simulink model "single_phase_inverter_rpid"  (R2020a)
settings: Solver=VariableStepAuto  StartTime=0.0  StopTime=simlength  RelTol=1e-3
undefined symbols (not defined in the file): A, Aed, Aresd, B, Bed, Bresd, C, Ce, Cres, d, E, ki, kp, Led, simlength, Tc, Ts, w, w0
settings Model: Creator=dbagn  LastModifiedBy=dabagnara
settings DataIOCC: ReturnWorkspaceOutputs=off

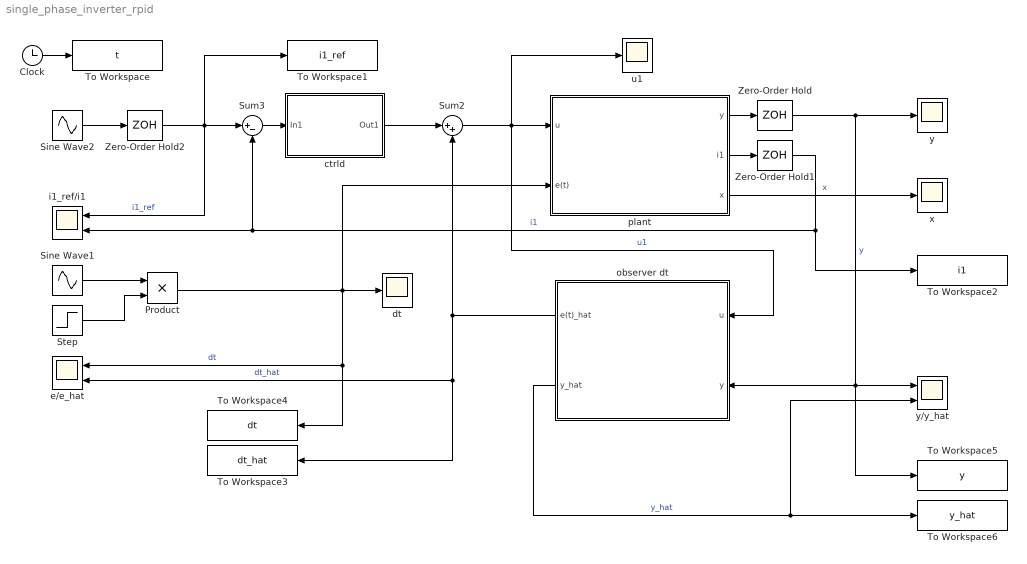
== system single_phase_inverter_rpid ==
  Clock : Clock
  Product : Product
  Sine Wave1 : Sin  Amplitude=d  Frequency=w  SampleTime=0
  Sine Wave2 : Sin  Amplitude=20  Frequency=w0  SampleTime=0
  Step : Step  Time=simlength/2  SampleTime=0
  Sum2 : Sum  Inputs=|++
  Sum3 : Sum  Inputs=|+-
  To Workspace : ToWorkspace  VariableName=t  SampleTime=Tc
      settings: MaxDataPoints=Nc
  To Workspace1 : ToWorkspace  VariableName=i1_ref  SampleTime=Tc
      settings: MaxDataPoints=Nc
  To Workspace2 : ToWorkspace  VariableName=i1  SampleTime=Tc
      settings: MaxDataPoints=Nc
  To Workspace3 : ToWorkspace  VariableName=dt_hat  SampleTime=Tc
      settings: MaxDataPoints=Nc
  To Workspace4 : ToWorkspace  VariableName=dt  SampleTime=Tc
      settings: MaxDataPoints=Nc
  To Workspace5 : ToWorkspace  VariableName=y  SampleTime=Tc
      settings: MaxDataPoints=Nc
  To Workspace6 : ToWorkspace  VariableName=y_hat  SampleTime=Tc
      settings: MaxDataPoints=Nc
  Zero-Order Hold : ZeroOrderHold  SampleTime=Ts
  Zero-Order Hold1 : ZeroOrderHold  SampleTime=Ts
  Zero-Order Hold2 : ZeroOrderHold  SampleTime=Ts
  ctrld : Subsystem
  dt : Scope
  e/e_hat : Scope  NumInputPorts=2
  i1_ref/i1 : Scope  NumInputPorts=2
  observer dt : Subsystem
  "plant " : Subsystem
  u1 : Scope
  x : Scope
  y : Scope
  y/y_hat : Scope  NumInputPorts=2
  wires:
  observer dt/2(y_hat) -> To Workspace6/1, y/y_hat/2  "y_hat"
  "plant "/1(y) -> Zero-Order Hold/1
  Product/1 -> To Workspace4/1, e/e_hat/1, dt/1, "plant "/2(e(t))  "dt"
  Sine Wave2/1 -> Zero-Order Hold2/1
  ctrld/1(Out1) -> Sum2/1
  Sum2/1 -> observer dt/1(u), "plant "/1(u), u1/1  "u1"
  "plant "/2(i1) -> Zero-Order Hold1/1
  "plant "/3(x) -> x/1  "x"
  Sum3/1 -> ctrld/1(In1)
  observer dt/1(e(t)_hat) -> Sum2/2, To Workspace3/1, e/e_hat/2  "dt_hat"
  Zero-Order Hold/1 -> To Workspace5/1, observer dt/2(y), y/y_hat/1, y/1  "y"
  Zero-Order Hold1/1 -> To Workspace2/1, Sum3/2, i1_ref/i1/2  "i1"
  Zero-Order Hold2/1 -> To Workspace1/1, Sum3/1, i1_ref/i1/1  "i1_ref"
  Sine Wave1/1 -> Product/1
  Step/1 -> Product/2
  Clock/1 -> To Workspace/1

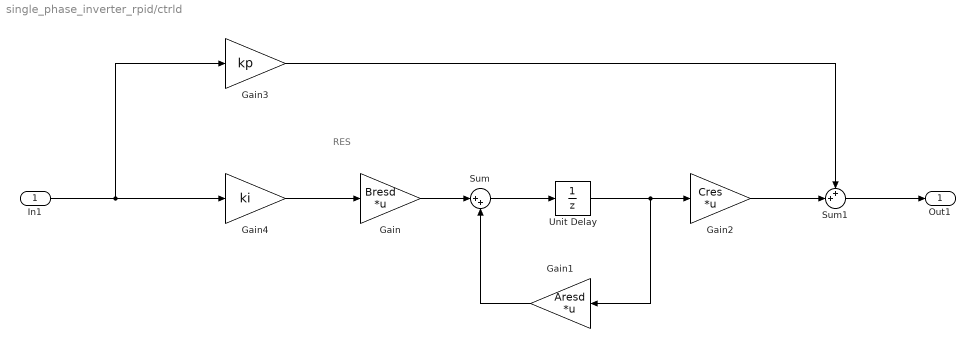
== system single_phase_inverter_rpid/ctrld ==
  note: RES
  In1 : Inport
  Gain : Gain  Gain=Bresd  Multiplication=Matrix(K*u)
  Gain1 : Gain  Gain=Aresd  Multiplication=Matrix(K*u)
  Gain2 : Gain  Gain=Cres  Multiplication=Matrix(K*u)
  Gain3 : Gain  Gain=kp
  Gain4 : Gain  Gain=ki
  Sum : Sum  Inputs=|++
  Sum1 : Sum  Inputs=++|
  Unit Delay : UnitDelay  SampleTime=Ts  HasFrameUpgradeWarning=on
  Out1 : Outport
  wires:
  In1/1 -> Gain4/1, Gain3/1
  Sum/1 -> Unit Delay/1
  Gain/1 -> Sum/1
  Gain1/1 -> Sum/2
  Unit Delay/1 -> Gain2/1, Gain1/1
  Gain4/1 -> Gain/1
  Gain2/1 -> Sum1/2
  Sum1/1 -> Out1/1
  Gain3/1 -> Sum1/1

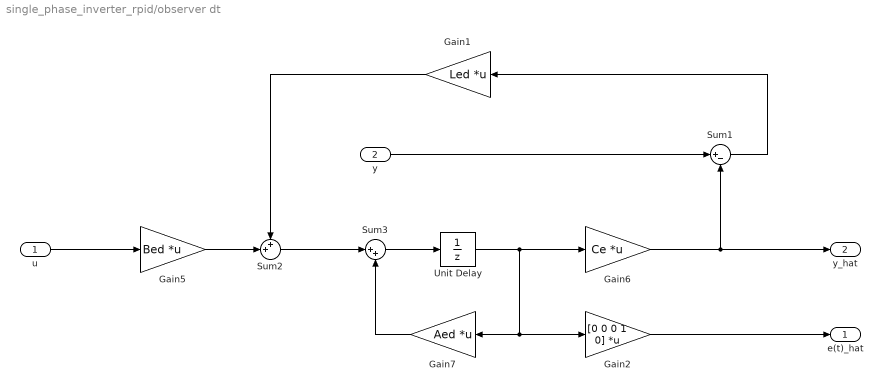
== system single_phase_inverter_rpid/observer dt ==
  u : Inport
  y : Inport  Port=2
  Gain1 : Gain  Gain=Led  Multiplication=Matrix(K*u)
  Gain2 : Gain  Gain=[0 0 0 1 0]  Multiplication=Matrix(K*u)
  Gain5 : Gain  Gain=Bed  Multiplication=Matrix(K*u)
  Gain6 : Gain  Gain=Ce  Multiplication=Matrix(K*u)
  Gain7 : Gain  Gain=Aed  Multiplication=Matrix(K*u)
  Sum1 : Sum  Inputs=|+-
  Sum2 : Sum  Inputs=++|
  Sum3 : Sum  Inputs=|++
  Unit Delay : UnitDelay  SampleTime=Ts  HasFrameUpgradeWarning=on
  e(t)_hat : Outport
  y_hat : Outport  Port=2
  wires:
  Sum2/1 -> Sum3/1
  Gain7/1 -> Sum3/2
  Gain6/1 -> y_hat/1, Sum1/2
  Sum1/1 -> Gain1/1
  u/1 -> Gain5/1
  Gain1/1 -> Sum2/1
  Gain5/1 -> Sum2/2
  y/1 -> Sum1/1
  Gain2/1 -> e(t)_hat/1
  Sum3/1 -> Unit Delay/1
  Unit Delay/1 -> Gain6/1, Gain2/1, Gain7/1

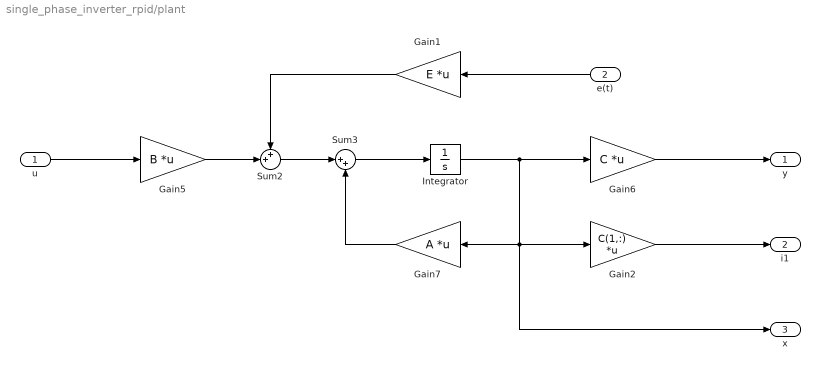
== system single_phase_inverter_rpid/plant  ==
  u : Inport
  e(t) : Inport  Port=2
  Gain1 : Gain  Gain=E  Multiplication=Matrix(K*u)
  Gain2 : Gain  Gain=C(1,:)  Multiplication=Matrix(K*u)
  Gain5 : Gain  Gain=B  Multiplication=Matrix(K*u)
  Gain6 : Gain  Gain=C  Multiplication=Matrix(K*u)
  Gain7 : Gain  Gain=A  Multiplication=Matrix(K*u)
  Integrator : Integrator
  Sum2 : Sum  Inputs=++|
  Sum3 : Sum  Inputs=|++
  y : Outport
  i1 : Outport  Port=2
  x : Outport  Port=3
  wires:
  Sum3/1 -> Integrator/1
  Gain5/1 -> Sum2/2
  Gain1/1 -> Sum2/1
  Gain7/1 -> Sum3/2
  u/1 -> Gain5/1
  Sum2/1 -> Sum3/1
  Gain6/1 -> y/1
  e(t)/1 -> Gain1/1
  Integrator/1 -> x/1, Gain2/1, Gain7/1, Gain6/1
  Gain2/1 -> i1/1
